simulink library "INT_InjCrv_MI1SOEAirMsCor"  (R2016b)
settings: Solver=VariableStepAuto  StartTime=0.0  StopTime=10.0  RelTol=1e-3
settings Model: Creator=Administrator  LastModifiedBy=Administrator

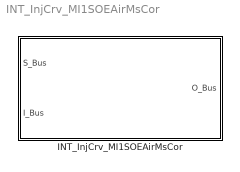
== system INT_InjCrv_MI1SOEAirMsCor ==
  INT_InjCrv_MI1SOEAirMsCor : Subsystem

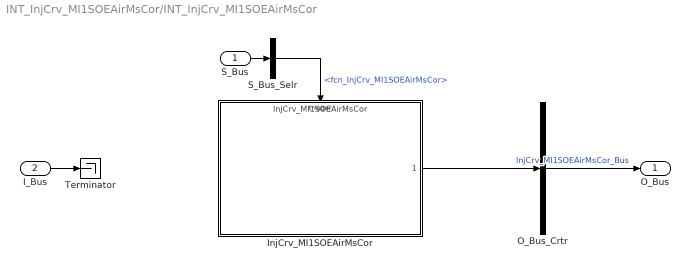
== system INT_InjCrv_MI1SOEAirMsCor/INT_InjCrv_MI1SOEAirMsCor ==
  S_Bus : Inport
  I_Bus : Inport  Port=2
  InjCrv_MI1SOEAirMsCor : ModelReference  ModelNameDialog=InjCrv_MI1SOEAirMsCor  SimulationMode=Normal  ModelReferenceVersion=1.5  TriggerPortName=function  TriggerPortTriggerType=function-call  TriggerPortStatesWhenEnabling=held
  O_Bus_Crtr : BusCreator  Inputs=1
  S_Bus_Selr : BusSelector  OutputSignals=fcn_InjCrv_MI1SOEAirMsCor
  Terminator : Terminator
  O_Bus : Outport
  wires:
  S_Bus_Selr/1 -> InjCrv_MI1SOEAirMsCor/Trigger  "<fcn_InjCrv_MI1SOEAirMsCor>"
  S_Bus/1 -> S_Bus_Selr/1
  I_Bus/1 -> Terminator/1
  O_Bus_Crtr/1 -> O_Bus/1  "InjCrv_MI1SOEAirMsCor_Bus"
  InjCrv_MI1SOEAirMsCor/1 -> O_Bus_Crtr/1
